simulink model "bio_matfunc_skew"  (R2017b)
settings: Solver=VariableStepAuto  StartTime=0.0  StopTime=10.0  RelTol=1e-3
settings Model: Creator=ktrinh  LastModifiedBy=hbourbou

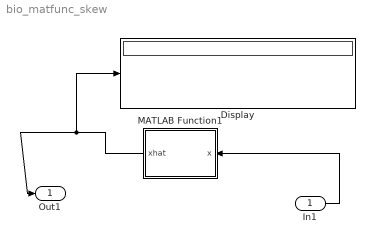
== system bio_matfunc_skew ==
  In1 : Inport  OutDataTypeStr=double  PortDimensions=3
  Display : Display
  MATLAB Function1 : MATLAB Function  TreatAsAtomicUnit=on
  Out1 : Outport
  wires:
  In1/1 -> MATLAB Function1/1(x)
  MATLAB Function1/1(xhat) -> Display/1, Out1/1

== matlab function bio_matfunc_skew/MATLAB Function1 ==
  data: x input; xhat output
function xhat = skew(x)
% Computes the hat map, mapping a 3-vector into a 3X3 skew-symmetric matrix
xhat = [  0   -x(3)  x(2)
         x(3)   0   -x(1)
        -x(2)  x(1)  0];
